simulink model "PR_planningsim_2joint"  (R2024a)
settings: Solver=ode45  StartTime=0.0  StopTime=stoptime
undefined symbols (not defined in the file): amp_factor, arm_radius, arm_radius_previus, begintime, controlactivate, damping_coeff, I_est, ifreskicking, ifreslosetrack, ifresnoise, ifrobotkicking, ifrobotnoise, ini_theta_p, ini_thetadot_p, pendepth, penlength, penposx, penposz, penrho, penwidth, rc, res_kick_height, res_kick_period, res_kick_start, res_losetrack_period, res_losetrack_start, res_noise_seed, res_noise_variance, robot_kick_height, robot_kick_period, robot_kick_start, robot_noise_seed, robot_noise_variance, robot_pendepth, robot_penlength, robot_penwidth, robot_pulse_freq, robot_pulse_hight, robot_pulse_period, robot_pulse_start, robot_sphere_mass, samplingrate, sphere_mass, sphere_radius, spring_position_scale, switch_threshold, torquelim, Win, X, Y, Z
libraries: sm_lib x25, nesl_utility x11, dspindex x5
(part 2 of 2)

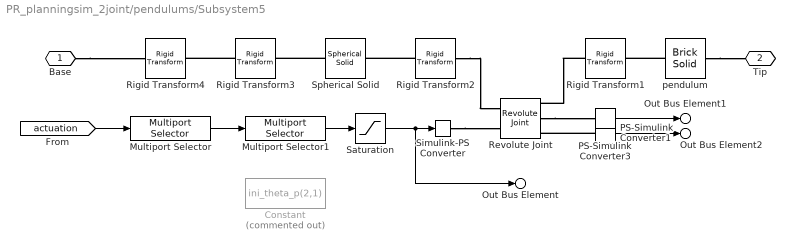
== system PR_planningsim_2joint/pendulums/Subsystem5 ==
  Constant : Constant  Commented=on  Value=ini_theta_p(2,1)
  Multiport Selector : dspindex/Multiport Selector  rowsOrCols=Rows  idxCellArray=pendulum_label(1)  idxErrMode=Clip Index
  Multiport Selector1 : dspindex/Multiport Selector  rowsOrCols=Columns  idxCellArray=pendulum_label(2)  idxErrMode=Clip Index
  PS-Simulink Converter1 : nesl_utility/PS-Simulink Converter  PhysicalDomain=network_engine_domain  SubClassName=ps_output  LeftPortType=input  RightPortType=output  PseudoPeriodic=off  Frequencies=[]  VectorFormat=1-D array  Unit=1  AffineConversion=off
  PS-Simulink Converter3 : nesl_utility/PS-Simulink Converter  PhysicalDomain=network_engine_domain  SubClassName=ps_output  LeftPortType=input  RightPortType=output  PseudoPeriodic=off  Frequencies=[]  VectorFormat=1-D array  Unit=1  AffineConversion=off
  Revolute Joint : sm_lib/Joints/Revolute Joint  JointMode=Normal  CompositeWrenchDir=FollowerOnBase  CompositeWrenchFrame=BaseFrame  SenseConstraintForce=off  SenseConstraintTorque=off  SenseTotalForce=off  SenseTotalTorque=off  PositionTargetSpecify=on  PositionTargetPriority=High  PositionTargetValue=ini_theta_p(pendulum_label(1), pendulum_label(2))  PositionTargetValueUnits=rad  VelocityTargetSpecify=on  VelocityTargetPriority=High  VelocityTargetValue=ini_thetadot_p(pendulum_label(1), pendulum_label(2))  VelocityTargetValueUnits=rad/s  EquilibriumPosition=0  EquilibriumPositionUnits=rad  SpringStiffness=0  SpringStiffnessUnits=N*m/rad  DampingCoefficient=damping_coeff(pendulum_label(1), pendulum_label(2))  DampingCoefficientUnits=N*m/(rad/s)  LowerLimitSpecify=off  LowerLimitBound=-90  LowerLimitBoundUnits=deg  LowerLimitStiffness=1e4  LowerLimitStiffnessUnits=N*m/deg  LowerLimitDamping=10  LowerLimitDampingUnits=N*m/(deg/s)  LowerLimitTransitionRegionWidth=0.1  LowerLimitTransitionRegionWidthUnits=deg  UpperLimitSpecify=off  UpperLimitBound=90  UpperLimitBoundUnits=deg  UpperLimitStiffness=1e4  UpperLimitStiffnessUnits=N*m/deg  UpperLimitDamping=10  UpperLimitDampingUnits=N*m/(deg/s)  UpperLimitTransitionRegionWidth=0.1  UpperLimitTransitionRegionWidthUnits=deg  TorqueActuationMode=ComputedTorque  MotionActuationMode=InputMotion  SensePosition=on  SenseVelocity=on  SenseAcceleration=off  SenseTorqueForce=off  SenseLowerLimitTorqueForce=off  SenseUpperLimitTorqueForce=off
  Rigid Transform1 : sm_lib/Frames and Transforms/Rigid Transform  RotationMethod=AlignedAxes  FollAlignAxisA=+X  BaseAlignAxisA=+X  FollAlignAxisB=-Z  BaseAlignAxisB=+Y  RotationStandardAxis=+Z  RotationAngle=180  RotationAngleUnits=deg  RotationArbitraryAxis=[0 0 1]  RotationSequenceAxes=FollowerAxes  RotationSequence=XYX  RotationSequenceAngles=[0 0 0]  RotationSequenceAnglesUnits=deg  RotationMatrix=[1 0 0; 0 1 0; 0 0 1]  Quaternion=[1 0 0 0]  TranslationMethod=None  TranslationCartesianOffset=[arm_radius*spring_position_scale 0 0]  TranslationCartesianOffsetUnits=m  TranslationStandardAxis=+Z  TranslationStandardOffset=0  TranslationStandardOffsetUnits=m  TranslationROffset=arm_radius_previus*spring_position_scale  TranslationROffsetUnits=m  TranslationThetaOffset=theta  TranslationThetaOffsetUnits=deg  TranslationZOffset=0  TranslationZOffsetUnits=m
  Rigid Transform2 : sm_lib/Frames and Transforms/Rigid Transform  RotationMethod=AlignedAxes  FollAlignAxisA=+X  BaseAlignAxisA=+X  FollAlignAxisB=+Y  BaseAlignAxisB=+Z  RotationStandardAxis=+Z  RotationAngle=180  RotationAngleUnits=deg  RotationArbitraryAxis=[0 0 1]  RotationSequenceAxes=FollowerAxes  RotationSequence=XYX  RotationSequenceAngles=[0 0 0]  RotationSequenceAnglesUnits=deg  RotationMatrix=[1 0 0; 0 1 0; 0 0 1]  Quaternion=[1 0 0 0]  TranslationMethod=None  TranslationCartesianOffset=[arm_radius*spring_position_scale 0 0]  TranslationCartesianOffsetUnits=m  TranslationStandardAxis=+Z  TranslationStandardOffset=0  TranslationStandardOffsetUnits=m  TranslationROffset=arm_radius_previus*spring_position_scale  TranslationROffsetUnits=m  TranslationThetaOffset=theta  TranslationThetaOffsetUnits=deg  TranslationZOffset=0  TranslationZOffsetUnits=m
  Rigid Transform3 : sm_lib/Frames and Transforms/Rigid Transform  RotationMethod=None  FollAlignAxisA=+X  BaseAlignAxisA=+X  FollAlignAxisB=+Y  BaseAlignAxisB=+Z  RotationStandardAxis=+Z  RotationAngle=180  RotationAngleUnits=deg  RotationArbitraryAxis=[0 0 1]  RotationSequenceAxes=FollowerAxes  RotationSequence=XYX  RotationSequenceAngles=[0 0 0]  RotationSequenceAnglesUnits=deg  RotationMatrix=[1 0 0; 0 1 0; 0 0 1]  Quaternion=[1 0 0 0]  TranslationMethod=StandardAxis  TranslationCartesianOffset=[arm_radius*spring_position_scale 0 0]  TranslationCartesianOffsetUnits=m  TranslationStandardAxis=+X  TranslationStandardOffset=penposx(pendulum_label(1), pendulum_label(2))  TranslationStandardOffsetUnits=m  TranslationROffset=arm_radius_previus*spring_position_scale  TranslationROffsetUnits=m  TranslationThetaOffset=theta  TranslationThetaOffsetUnits=deg  TranslationZOffset=0  TranslationZOffsetUnits=m
  Rigid Transform4 : sm_lib/Frames and Transforms/Rigid Transform  RotationMethod=None  FollAlignAxisA=+X  BaseAlignAxisA=+X  FollAlignAxisB=+Y  BaseAlignAxisB=+Z  RotationStandardAxis=+Z  RotationAngle=180  RotationAngleUnits=deg  RotationArbitraryAxis=[0 0 1]  RotationSequenceAxes=FollowerAxes  RotationSequence=XYX  RotationSequenceAngles=[0 0 0]  RotationSequenceAnglesUnits=deg  RotationMatrix=[1 0 0; 0 1 0; 0 0 1]  Quaternion=[1 0 0 0]  TranslationMethod=StandardAxis  TranslationCartesianOffset=[arm_radius*spring_position_scale 0 0]  TranslationCartesianOffsetUnits=m  TranslationStandardAxis=+Z  TranslationStandardOffset=penposz(pendulum_label(1), pendulum_label(2))  TranslationStandardOffsetUnits=m  TranslationROffset=arm_radius_previus*spring_position_scale  TranslationROffsetUnits=m  TranslationThetaOffset=theta  TranslationThetaOffsetUnits=deg  TranslationZOffset=0  TranslationZOffsetUnits=m
  Saturation : Saturate  UpperLimit=pi/2  LowerLimit=-pi/2
  Simulink-PS Converter : nesl_utility/Simulink-PS Converter  PhysicalDomain=network_engine_domain  SubClassName=ps_input  LeftPortType=input  RightPortType=output  PseudoPeriodic=off  Frequencies=[]  NoiseDistribution=none  NoiseParameters=[]  Unit=1  AffineConversion=off  FilteringAndDerivatives=filter  SimscapeFilterOrder=2  InputFilterTimeConstant=0.05  UdotUserProvided=0
  Spherical Solid : sm_lib/Body Elements/Spherical Solid  SphereRadius=sphere_radius(pendulum_label(1), pendulum_label(2))  SphereRadiusUnits=m  ExportEntireGeometry=off  InertiaType=CalculateFromGeometry  BasedOnType=Mass  Density=1000  DensityUnits=kg/m^3  Mass=sphere_mass(pendulum_label(1), pendulum_label(2))  MassUnits=kg  CenterOfMass=[0 0 0]  CenterOfMassUnits=m  MomentsOfInertia=[1 1 1]  MomentsOfInertiaUnits=kg*m^2  ProductsOfInertia=[0 0 0]  ProductsOfInertiaUnits=kg*m^2  GraphicType=FromGeometry  MarkerShape=Sphere  MarkerSize=10  GraphicVisPropType=SimpleVisualProperties  GraphicDiffuseColor=[0.6 0.6 0.6]  GraphicOpacity=1.0  GraphicSpecularColor=[0.5 0.5 0.5 1.0]  GraphicAmbientColor=[0.15 0.15 0.15 1.0]  GraphicEmissiveColor=[0.0 0.0 0.0 1.0]  GraphicShininess=75  DoExposeReferenceFrame=on  SerializedFrames=<Frames><Frame><Id>Frame1</Id><Value><Name>F1</Name><Origin><Source>ReferenceFrame</Source><FeatureName></FeatureName></Origin><PrimaryAxis><DefinedDirection>+Z</DefinedDirection><Source>ReferenceFrame</Source><SourceDirection>+Z</SourceDirection><FeatureName></FeatureName></PrimaryAxis><SecondaryAxis><DefinedDirection>+X</DefinedDirection><Source>ReferenceFrame</Source><SourceDirection>+X</SourceDirection><FeatureName></FeatureName></SecondaryAxis></Value></Frame></Frames>
  pendulum : sm_lib/Body Elements/Brick Solid  BrickDimensions=[penwidth(pendulum_label(1), pendulum_label(2)) pendepth(pendulum_label(1), pendulum_label(2)) penlength(pendulum_label(1), pendulum_label(2))]  BrickDimensionsUnits=m  ExportEntireGeometry=off  InertiaType=CalculateFromGeometry  BasedOnType=Density  Density=penrho(pendulum_label(1), pendulum_label(2))  DensityUnits=kg/m^3  Mass=1  MassUnits=kg  CenterOfMass=[0 0 0]  CenterOfMassUnits=m  MomentsOfInertia=[1 1 1]  MomentsOfInertiaUnits=kg*m^2  ProductsOfInertia=[0 0 0]  ProductsOfInertiaUnits=kg*m^2  GraphicType=FromGeometry  MarkerShape=Sphere  MarkerSize=10  GraphicVisPropType=SimpleVisualProperties  GraphicDiffuseColor=[1.0 0.0 0.0]  GraphicOpacity=1.0  GraphicSpecularColor=[0.5 0.5 0.5 1.0]  GraphicAmbientColor=[0.15 0.15 0.15 1.0]  GraphicEmissiveColor=[0.0 0.0 0.0 1.0]  GraphicShininess=75  DoExposeReferenceFrame=off  SerializedFrames=<Frames><Frame><Id>Frame1</Id><Value><Name>F1</Name><Origin><Source>GeometricFeature</Source><FeatureName>-z surface</FeatureName></Origin><PrimaryAxis><DefinedDirection>+Z</DefinedDirection><Source>ReferenceFrame</Source><SourceDirection>+Z</SourceDirection><FeatureName></FeatureName></PrimaryAxis><SecondaryAxis><DefinedDirection>+X</DefinedDirection><Source>ReferenceFrame</Source><SourceDirection>+X</SourceDirection><FeatureName></FeatureName></SecondaryAxis></Value></Frame><Frame><Id>Frame2</Id><Value><Name>F2</Name><Origin><Source>GeometricFeature</Source><FeatureName>+z surface</FeatureName></Origin><PrimaryAxis><DefinedDirection>+Z</DefinedDirection><Source>ReferenceFrame</Source><SourceDirection>-Z</SourceDirection><FeatureName></FeatureName></PrimaryAxis><SecondaryAxis><DefinedDirection>+X</DefinedDirection><Source>ReferenceFrame</Source><SourceDirection>+X</SourceDirection><FeatureName></FeatureName></SecondaryAxis></Value></Frame></Frames>
  Base : PMIOPort  Side=Left
  Tip : PMIOPort  Port=2  Side=Right
  Out Bus Element : Outport  PortName=out  Element=torque
  Out Bus Element1 : Outport  PortName=out  Element=theta
  Out Bus Element2 : Outport  PortName=out  Element=thetadot
  wires:
  PS-Simulink Converter3/1 -> Out Bus Element1/1
  PS-Simulink Converter1/1 -> Out Bus Element2/1
  Multiport Selector/1 -> Multiport Selector1/1
  Saturation/1 -> Simulink-PS Converter/1, Out Bus Element/1
  [actuation] -> Multiport Selector/1
  Multiport Selector1/1 -> Saturation/1
  connections:
  Spherical Solid/LConn1 -- Rigid Transform3/RConn1
  Rigid Transform1/LConn1 -- Revolute Joint/RConn1
  Rigid Transform2/RConn1 -- Revolute Joint/LConn1
  pendulum/RConn1 -- Tip/RConn1
  PS-Simulink Converter1/LConn1 -- Revolute Joint/RConn3
  pendulum/LConn1 -- Rigid Transform1/RConn1
  Rigid Transform2/LConn1 -- Spherical Solid/RConn1
  Revolute Joint/RConn2 -- PS-Simulink Converter3/LConn1
  Base/RConn1 -- Rigid Transform4/LConn1
  Rigid Transform3/LConn1 -- Rigid Transform4/RConn1
  Simulink-PS Converter/RConn1 -- Revolute Joint/LConn2

== system PR_planningsim_2joint/Floor Surface/Floor/Grid ==
  Mesh XY-Y : sm_lib/Body Elements/Extruded Solid  Commented=on  ExtrusionType=General  PolygonNumSides=3  PolygonOuterRadius=1  PolygonOuterRadiusUnits=m  ExportEntireGeometry=off  ExtrusionCrossSection=mesh_xsec  ExtrusionCrossSectionUnits=m  ExportConvexHullGeometry=off  ExtrusionLength=grid_linewidth  ExtrusionLengthUnits=m  InertiaType=CalculateFromGeometry  BasedOnType=Density  Density=1000  DensityUnits=kg/(m^3)  Mass=1  MassUnits=kg  CenterOfMass=[0 0 0]  CenterOfMassUnits=m  MomentsOfInertia=[1 1 1]  MomentsOfInertiaUnits=kg*m^2  ProductsOfInertia=[0 0 0]  ProductsOfInertiaUnits=kg*m^2  GraphicType=FromGeometry  MarkerShape=Sphere  MarkerSize=10  GraphicVisPropType=SimpleVisualProperties  GraphicDiffuseColor=[0.5 0.5 0.5]  GraphicOpacity=1.0  GraphicSpecularColor=[0.5 0.5 0.5 1.0]  GraphicAmbientColor=[0.15 0.15 0.15 1.0]  GraphicEmissiveColor=[0.0 0.0 0.0 1.0]  GraphicShininess=75  DoExposeReferenceFrame=on  SerializedFrames=<Frames/>
  R : PMIOPort  Side=Left
  connections:
  R/RConn1 -- Mesh XY-Y/RConn1

== matlab function PR_planningsim_2joint/Actuation/Subsystem1/MATLAB Function ==
  data: k11 input; k12 input; y output; k21 input; k22 input
function y = fcn(k11, k12, k21, k22)

y = zeros(2,2);

y(1,2) = y(1,2) + k11 + k12;
y(2,2) = y(2,2) + k21 + k22;

end

== matlab function PR_planningsim_2joint/Actuation/inputs ==
  data: input input; act output; Win parameter; amp_factor parameter
function act = fcn(input, Win, amp_factor)

in = [input(1);
    input(2)];

in = amp_factor.*in;

inputmat = [in 0.*in];

act = Win*inputmat;

end

== matlab function PR_planningsim_2joint/readout/inputs ==
  data: s11 input; s21 input; const input; x input; output output size=3; Woutmat parameter
function output = fcn(s11, s21, const, x, Woutmat)

readoutt = [const; x; s11; s21];

output = Woutmat*readoutt;

end

== matlab function PR_planningsim_2joint/inputs ==
  data: PRinput output; Rout input; Routdelayed input; PRoutput input; iscontrol parameter; target output
function [PRinput,target] = fcn(Rout, Routdelayed, PRoutput, iscontrol)

if iscontrol
    PRinput = [Rout(1);
        Rout(2);
        PRoutput(2);
        PRoutput(3);];
    target = [PRoutput(1);
        PRoutput(2);
        PRoutput(3)];
else
    PRinput = [Routdelayed(1);
        Routdelayed(2);
        Rout(1);
        Rout(2)];
    target = [Routdelayed(3);
        Rout(1);
        Rout(2)];
end

end

== matlab function PR_planningsim_2joint/readout/MATLAB Function2 ==
  data: x input; altx1 output size=1; x1 input; x2 input; altx2 output size=1; numswitch output size=1
function [altx1, altx2, numswitch] = fcn(x, x1, x2)

altx1 = 2*pi*round((x(1)-x1)/2/pi) + x1;
altx2 = x2;

numswitch = abs((x(1)-x1) - 2*pi*round((x(1)-x1)/2/pi));

end

== matlab function PR_planningsim_2joint/readout/MATLAB Function ==
  data: u input; y1 output; y2 output; y3 output
function [y1, y2, y3] = fcn(u)

y1 = u(1);
y2 = u(2);
y3 = u(3);

end

== matlab function PR_planningsim_2joint/readout/MATLAB Function1 ==
  data: y1 input; u output; y2 input; y3 input
function u  = fcn(y1, y2, y3)

u = [y1; y2; y3];

end

== matlab function PR_planningsim_2joint/Actuation/Subsystem/MATLAB Function ==
  data: n1 input; n2 input; y output
function y = fcn(n1, n2)

y = zeros(4,1);

y(1,1) = y(1,1) + n1;
y(2,1) = y(2,1) + n2;

end
